simulink subsystem "IMU"  (R2023a)
settings: Solver=VariableStepAuto  StartTime=0.0  StopTime=10.0  RelTol=1e-3
undefined symbols (not defined in the file or in its folder): samplingTime
settings Model: Creator=JesseJabezArendse  LastModifiedBy=JesseJabezArendse

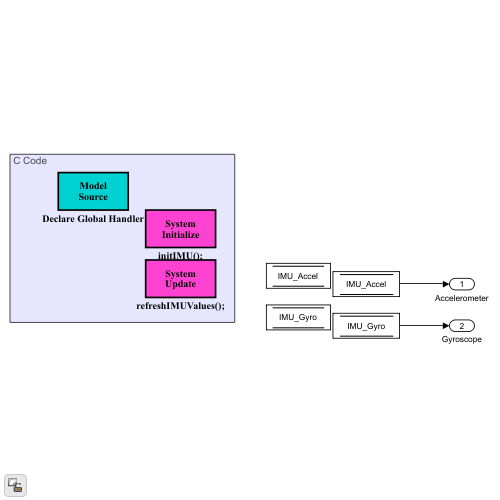
[thumbnail: Simulink's stored preview of the top-level diagram]
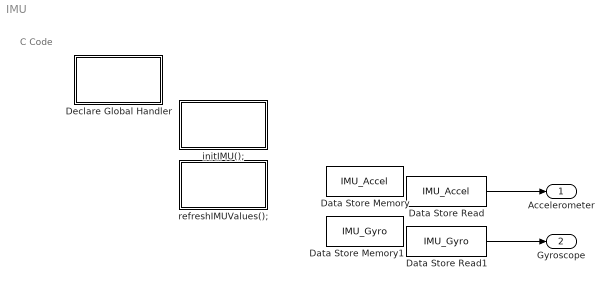
== system IMU ==
  note: C Code
  Data Store Memory : DataStoreMemory  DataStoreName=IMU_Accel  WriteAfterWriteMsg=warning  ShowAdditionalParam=off  OutDataTypeStr=single  Dimensions=3
  Data Store Memory1 : DataStoreMemory  DataStoreName=IMU_Gyro  WriteAfterWriteMsg=warning  ShowAdditionalParam=off  OutDataTypeStr=single  Dimensions=3
  Data Store Read : DataStoreRead  DataStoreName=IMU_Accel  SampleTime=samplingTime  IndexOptions=Index vector (dialog)  Indices=1  OutputSizes=1
  Data Store Read1 : DataStoreRead  DataStoreName=IMU_Gyro  SampleTime=samplingTime  IndexOptions=Index vector (dialog)  Indices=1  OutputSizes=1
  Declare Global Handler : Subsystem  TreatAsAtomicUnit=on  SystemSampleTime=samplingTime  mask(Model Source){ShowInLibBrowser=0}
      mask prompts: ShowInLibBrowser "Simulink:masks:CustCodeMaskParam1_MP"
      settings: CopyFcn=cccopyfcn(gcb)  OpenFcn=ccopenfcn('Model Source')
      mask Help: eval('feval(''rtwprivate'',''rtwhelpview'',''rtw_model_source_block'')');
      mask DialogControl ShowInLibBrowser Prompt: Mask Parameter 1:
      mask Display: disp('Model\nSource');
  initIMU(); : Subsystem  TreatAsAtomicUnit=on  SystemSampleTime=samplingTime  mask(System Initialize){ShowInLibBrowser=0}
      mask prompts: ShowInLibBrowser "Simulink:masks:CustCodeMaskParam1_MP"
      settings: CopyFcn=cccopyfcn(gcb)  OpenFcn=ccopenfcn('System Initialize Function')
      mask Help: eval('feval(''rtwprivate'',''rtwhelpview'',''rtw_sys_initialize_block'')');
      mask DialogControl ShowInLibBrowser Prompt: Mask Parameter 1:
      mask Display: disp('System\nInitialize');
  refreshIMUValues(); : Subsystem  TreatAsAtomicUnit=on  SystemSampleTime=samplingTime  mask(System Update){ShowInLibBrowser=0}
      mask prompts: ShowInLibBrowser "Simulink:masks:CustCodeMaskParam1_MP"
      settings: CopyFcn=cccopyfcn(gcb)  OpenFcn=ccopenfcn('System Update Function')
      mask Help: eval('feval(''rtwprivate'',''rtwhelpview'',''rtw_sys_update_block'')');
      mask DialogControl ShowInLibBrowser Prompt: Mask Parameter 1:
      mask Display: disp('System\nUpdate');
  Accelerometer : Outport  OutDataTypeStr=single  PortDimensions=3
  Gyroscope : Outport  Port=2  OutDataTypeStr=single  PortDimensions=3
  wires:
  Data Store Read1/1 -> Gyroscope/1
  Data Store Read/1 -> Accelerometer/1

== system IMU/Declare Global Handler ==

== system IMU/initIMU(); ==

== system IMU/refreshIMUValues(); ==
